simulink model "quad_3_ref_6_y_NN"  (R2018b)
settings: Solver=FixedStepAuto  StartTime=0.0  StopTime=options.T_train  FixedStep=0.01  RelTol=1e-3
undefined symbols (not defined in the file or in its folder): options
libraries: neural x70, simulink x3
(part 3 of 3)

== system quad_3_ref_6_y_NN/nn_1/Layer 3/Delays 1 ==
  "p{3}" : Inport  PortDimensions=30
      mask Display: e = 0.06;c1 = [120 230 180]/255;c2 = ([120 230 180]+0)/(256+128);c3 = ([120 230 180]+128)/(256+128);patch([0 1 1 0],[0 0 1 1],c1);patch([0 1 1 1-e 1-e 0+e],[0 0 1 1-e 0+e 0+e],c2);patch([0 0 1 1-e 0+e 0+e],[0 1 1 1-e 1-e 0+e],c3);plot([0 1 1 0 0],[0 0 1 1 0]);
  mux : Mux  Inputs=1
      mask Display: e = 0.06;c1 = [120 150 230]/255;c2 = ([120 150 230]+0)/383;c3 = ([120 150 230]+128)/383;patch([0 1 1 0],[0 0 1 1],c1);patch([0 1 1 1-e 1-e 0+e],[0 0 1 1-e 0+e 0+e],c2);patch([0 0 1 1-e 0+e 0+e],[0 1 1 1-e 1-e 0+e],c3);plot([0 1 1 0 0],[0 0 1 1 0]);disp('Mux')
  "pd{3,2}" : Outport
      mask Display: e = 0.06;c1 = [120 230 180]/255;c2 = ([120 230 180]+0)/(256+128);c3 = ([120 230 180]+128)/(256+128);patch([0 1 1 0],[0 0 1 1],c1);patch([0 1 1 1-e 1-e 0+e],[0 0 1 1-e 0+e 0+e],c2);patch([0 0 1 1-e 0+e 0+e],[0 1 1 1-e 1-e 0+e],c3);plot([0 1 1 0 0],[0 0 1 1 0]);
  wires:
  "p{3}"/1 -> mux/1
  mux/1 -> "pd{3,2}"/1

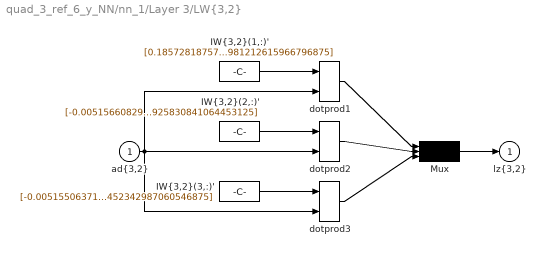
== system quad_3_ref_6_y_NN/nn_1/Layer 3/LW{3,2} ==
  "ad{3,2}" : Inport  PortDimensions=30
      mask Display: e = 0.06;c1 = [120 230 180]/255;c2 = ([120 230 180]+0)/(256+128);c3 = ([120 230 180]+128)/(256+128);patch([0 1 1 0],[0 0 1 1],c1);patch([0 1 1 1-e 1-e 0+e],[0 0 1 1-e 0+e 0+e],c2);patch([0 0 1 1-e 0+e 0+e],[0 1 1 1-e 1-e 0+e],c3);plot([0 1 1 0 0],[0 0 1 1 0]);
  "IW{3,2}(1,:)'" : Constant  Value=[0.1857281875784853042432587244547903537750244140625;0.277040190677199593682900058411178179085254669189453125;0.315494056537138245488449683762155473232269287109375;0.324866217035903737109236999458516947925090789794921875;-0.281775901414300256053735438399598933756351470947265625;-0.0639536564528310480515216340791084803640842437744140625;0.316096726125746130264815292321145534515380859375;0.177517209727092006854576311525306664407253265380859375;-0.269349930113234548034739646027446724474430084228515625;-0.210130833064223920825241975762764923274517059326171875;0.285428184999986511716230097590596415102481842041015625;-0.3025922272304171212198298235307447612285614013671875;0.0289653233236714206799700122019203263334929943084716796875;0.2941841193336862669838183137471787631511688232421875;0.291395800933710147351263231030316092073917388916015625;0.226631621301671193347004873430705629289150238037109375;0.139604264827299096030088776387856341898441314697265625;-0.0758165800260015287914683312919805757701396942138671875;-0.240037524438895089051726472462178207933902740478515625;0.2959677483582534573969269331428222358226776123046875;0.24137545844598273792058762410306371748447418212890625;0.278355272612209880822575769343529827892780303955078125;-0.15920426572792789610133468158892355859279632568359375;0.130647419351454685543245659573585726320743560791015625;-0.12156805028798485512897542548671481199562549591064453125;0.052706801430805770569687496163169271312654018402099609375;-0.11316435441703419362280413906773901544511318206787109375;-0.2691435382387485919508662846055813133716583251953125;0.29698744501262830386423274831031449139118194580078125;0.242057860586071871278335265742498449981212615966796875]
      mask Display: e = 0.06;c1 = [120 150 230]/255;c2 = ([120 150 230]+0)/383;c3 = ([120 150 230]+128)/383;patch([0 1 1 0],[0 0 1 1],c1);patch([0 1 1 1-e 1-e 0+e],[0 0 1 1-e 0+e 0+e],c2);patch([0 0 1 1-e 0+e 0+e],[0 1 1 1-e 1-e 0+e],c3);plot([0 1 1 0 0],[0 0 1 1 0]);disp('weights');
  "IW{3,2}(2,:)'" : Constant  Value=[-0.00515660829907267116711810928109116503037512302398681640625;-0.008543899139651194019062785400819848291575908660888671875;-0.01273981729703715405632724610995865077711641788482666015625;-0.01427174029188864323725027816180954687297344207763671875;0.0103380965396026140712404384203182416968047618865966796875;0.0016539869745993665724193011357101568137295544147491455078125;-0.0133143872862040886506651560239333775825798511505126953125;-0.005118097067021490191585098017412747140042483806610107421875;0.010188533397841460781396705215229303576052188873291015625;0.006843839782685100757431140294784199795685708522796630859375;-0.0107751584858007988521055864339359686709940433502197265625;0.0120062626637718050659486834774725139141082763671875;-0.00101804884713496452026959548931017707218416035175323486328125;-0.0116452965411331897660485168444211012683808803558349609375;-0.01125073174822936554473340464710418018512427806854248046875;-0.00707010558689995238790260145833599381148815155029296875;-0.003933690979214729370461167690109505201689898967742919921875;0.0014487562836469959105800686671727817156352102756500244140625;0.008078416176346712995748333696610643528401851654052734375;-0.01149165010160306359121573649417769047431647777557373046875;-0.00831945956633987036832333927804938866756856441497802734375;-0.0104121239080348544636667185159240034408867359161376953125;0.004593814793143898532468138995454864925704896450042724609375;-0.0037787393815741539271346738360080053098499774932861328125;0.003522810966000366854344871825333029846660792827606201171875;-0.0016569043005381979029311256823575604357756674289703369140625;0.00249813534490979372026941973672364838421344757080078125;0.0099900507162659531179560445934839663095772266387939453125;-0.01164387557702723126340504933295960654504597187042236328125;-0.007989091266656485335051485208168742246925830841064453125]
      mask Display: e = 0.06;c1 = [120 150 230]/255;c2 = ([120 150 230]+0)/383;c3 = ([120 150 230]+128)/383;patch([0 1 1 0],[0 0 1 1],c1);patch([0 1 1 1-e 1-e 0+e],[0 0 1 1-e 0+e 0+e],c2);patch([0 0 1 1-e 0+e 0+e],[0 1 1 1-e 1-e 0+e],c3);plot([0 1 1 0 0],[0 0 1 1 0]);disp('weights');
  "IW{3,2}(3,:)'" : Constant  Value=[-0.005155063717768811927533167960291393683291971683502197265625;-0.0085413495598970802513694167146240943111479282379150390625;-0.01273609387960667783945556408298216410912573337554931640625;-0.014267581120416920892335355119939777068793773651123046875;0.01033507397719002178504421607385665993206202983856201171875;0.0016534683543521036010182090336684268550015985965728759765625;-0.013310506296503855916402159209610545076429843902587890625;-0.00511656124374296715495713527843690826557576656341552734375;0.01018551606610077799042191060152617865242063999176025390625;0.006841813122156980252197566727545563480816781520843505859375;-0.01077199382499172651550534141051684855483472347259521484375;0.01200273950400643392655286589842944522388279438018798828125;-0.0010177514212246327636457454701712777023203670978546142578125;-0.01164189302697136128850186054251025780104100704193115234375;-0.0112474295669944789055616496398215531371533870697021484375;-0.00706801539323550186144640150587292737327516078948974609375;-0.003932498594961738279385254912767777568660676479339599609375;0.00144831289472373476480415721567851505824364721775054931640625;0.00807600697965458504123947847119779908098280429840087890625;-0.0114882761539536158712504487766636884771287441253662109375;-0.00831697874407414695918649982786519103683531284332275390625;-0.01040906690246597328386446434933532145805656909942626953125;0.00459243466862131917427536365039486554451286792755126953125;-0.0037776090486546505357867697938445417094044387340545654296875;0.0035217605717653859866145271695359042496420443058013916015625;-0.0016564100798328318386865021238918416202068328857421875;0.00249737753981014477810962404191741370595991611480712890625;0.00998711055350048719503330829638798604719340801239013671875;-0.0116404664102399031666568163245756295509636402130126953125;-0.00798674236609590859625740222327294759452342987060546875]
      mask Display: e = 0.06;c1 = [120 150 230]/255;c2 = ([120 150 230]+0)/383;c3 = ([120 150 230]+128)/383;patch([0 1 1 0],[0 0 1 1],c1);patch([0 1 1 1-e 1-e 0+e],[0 0 1 1-e 0+e 0+e],c2);patch([0 0 1 1-e 0+e 0+e],[0 1 1 1-e 1-e 0+e],c3);plot([0 1 1 0 0],[0 0 1 1 0]);disp('weights');
  Mux : Mux  Inputs=3
      mask Display: e = 0.06;c1 = [120 150 230]/255;c2 = ([120 150 230]+0)/383;c3 = ([120 150 230]+128)/383;patch([0 1 1 0],[0 0 1 1],c1);patch([0 1 1 1-e 1-e 0+e],[0 0 1 1-e 0+e 0+e],c2);patch([0 0 1 1-e 0+e 0+e],[0 1 1 1-e 1-e 0+e],c3);plot([0 1 1 0 0],[0 0 1 1 0]);disp('Mux');
  dotprod1 : neural/Weight Functions/dotprod
  dotprod2 : neural/Weight Functions/dotprod
  dotprod3 : neural/Weight Functions/dotprod
  "lz{3,2}" : Outport
      mask Display: e = 0.06;c1 = [120 230 180]/255;c2 = ([120 230 180]+0)/(256+128);c3 = ([120 230 180]+128)/(256+128);patch([0 1 1 0],[0 0 1 1],c1);patch([0 1 1 1-e 1-e 0+e],[0 0 1 1-e 0+e 0+e],c2);patch([0 0 1 1-e 0+e 0+e],[0 1 1 1-e 1-e 0+e],c3);plot([0 1 1 0 0],[0 0 1 1 0]);
  wires:
  "IW{3,2}(1,:)'"/1 -> dotprod1/1
  "ad{3,2}"/1 -> dotprod1/2, dotprod2/2, dotprod3/2
  dotprod1/1 -> Mux/1
  "IW{3,2}(2,:)'"/1 -> dotprod2/1
  dotprod2/1 -> Mux/2
  "IW{3,2}(3,:)'"/1 -> dotprod3/1
  dotprod3/1 -> Mux/3
  Mux/1 -> "lz{3,2}"/1

== matlab function quad_3_ref_6_y_NN/MATLAB Function ==
  data: r1 input; F output; r2 input; r3 input; x3 input; x6 input; x7 input; x8 input; x10 input; x11 input; tau_phi output; tau_theta output; tau_psi output
function [F,tau_phi,tau_theta,tau_psi] = fcn(r1,r2,r3,x3,x6,x7,x8,x10,x11)
%initialization
m=1.4;
g=9.81;
F= m*g-10*(x3-r1)+3*x6;
tau_phi=-(x7-r2)-x10;
tau_theta=-(x8-r3)-x11;
tau_psi=0;
